simulink model "channel_rayleigh"  (R2020a)
settings: Solver=ode45  StartTime=0.0  StopTime=10.0  RelTol=1e-3  EnableMultiTasking=on
libraries: commdigbbndpm3 x2, commsink2 x1
settings Model: Creator=Csurgai  LastModifiedBy=L.Csurgai
settings DataIOCC: LimitDataPoints=on  SaveFormat=Array  SignalLoggingSaveFormat=ModelDataLogs  ReturnWorkspaceOutputs=off
settings OptimizationCC: InitFltsAndDblsToZero=on  LifeSpan=inf
settings DebuggingCC: SaveWithParameterizedLinksMsg=none  UnderspecifiedInitializationDetection=Classic  MergeDetectMultiDrivingBlocksExec=none  SignalResolutionControl=TryResolveAllWithWarning  SolverPrmCheckMsg=warning  MultiTaskDSMMsg=warning  MultiTaskCondExecSysMsg=none  FcnCallInpInsideContextMsg=warning  SFUnexpectedBacktrackingDiag=warning  SFNoUnconditionalDefaultTransitionDiag=warning  SFExecutionAtInitializationDiag=none  ArithmeticOperatorsInVariantConditions=warning
settings HardwareCC: ProdBitPerPointer=32  ProdBitPerSizeT=32  ProdBitPerPtrDiffT=32  ProdLargestAtomicFloat=None  ProdIntDivRoundTo=Undefined  ProdEndianess=Unspecified  ProdWordSize=32  ProdHWDeviceType=32-bit Generic
settings ModelReferenceCC: PropagateSignalLabelsOutOfModel=off
settings SFSimCC: SimUseLocalCustomCode=off  CustomCodeUndefinedFunction=UseInterfaceOnly
settings RTWCC: RTWUseLocalCustomCode=off
settings CodeAppCC: StateflowObjectComments=on
settings GRTTargetCC: TargetFcnLib=ansi_tfl_tmw.mat  TargetLangStandard=C89/C90 (ANSI)  CombineOutputUpdateFcns=off  GRTInterface=on
settings ConfigComp: CovMetricSettings=dw  CovHtmlReporting=on  CovSaveCumulativeToWorkspaceVar=on  CovSaveSingleToWorkspaceVar=on  CovExternalEMLEnable=off

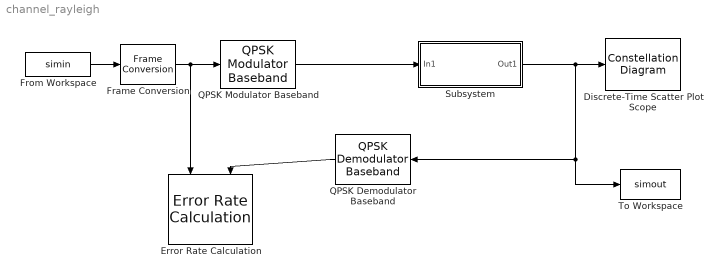
== system channel_rayleigh ==
  Discrete-Time Scatter Plot Scope : ConstellationDiagram  Tag=ScatterPlot
  Error Rate Calculation : commsink2/Error Rate Calculation  N=0  st_delay=0  cp_mode=Entire frame  subframe=[]  PMode=Workspace  WsName=ErrorVec  RsMode2=off  stop=off  numErr=100  maxBits=1e6
  Frame Conversion : FrameConversion
  From Workspace : FromWorkspace  VariableName=simin  SampleTime=1e-3
  QPSK Demodulator Baseband : commdigbbndpm3/QPSK Demodulator Baseband  OutType=Integer  DecType=Hard decision  VarSource=Dialog  Variance=1  Dec=Binary  Ph=pi/4  outDtype1=double  outDtype2=double  derotateFactorWordLen=16  derotateFactorDataTypeStr=Inherit: Same word length as input  derotateFactorLastDataTypeStr=Inherit: Same word length as input
  QPSK Modulator Baseband : commdigbbndpm3/QPSK Modulator Baseband  InType=Integer  Enc=Binary  Ph=pi/4  outDtype=double  outWordLen=16  outUDDataType=sfix(16)  outFracLenMode=Best precision  outFracLen=15  outDataTypeStr=double  outLastDataTypeStr=double
  Subsystem : Subsystem
  To Workspace : ToWorkspace  VariableName=simout  SaveFormat=Structure  SampleTime=-1
      settings: Save2DSignal=2-D array (concatenate along first dimension)
  wires:
  From Workspace/1 -> Frame Conversion/1
  Frame Conversion/1 -> QPSK Modulator Baseband/1, Error Rate Calculation/1
  QPSK Demodulator Baseband/1 -> Error Rate Calculation/2
  QPSK Modulator Baseband/1 -> Subsystem/1(In1)
  Subsystem/1(Out1) -> Discrete-Time Scatter Plot Scope/1, To Workspace/1, QPSK Demodulator Baseband/1

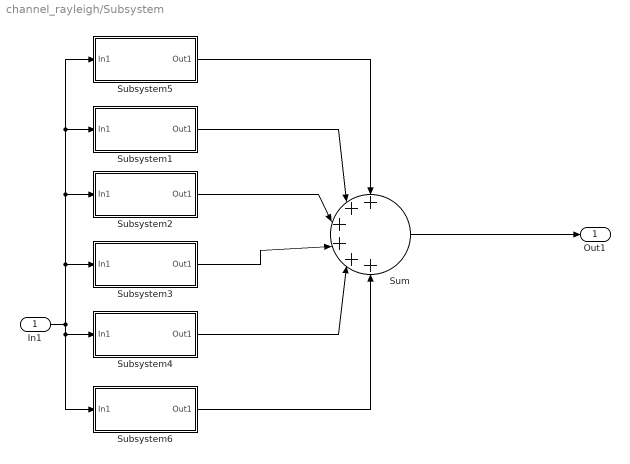
== system channel_rayleigh/Subsystem ==
  In1 : Inport
  Subsystem1 : Subsystem
  Subsystem2 : Subsystem
  Subsystem3 : Subsystem
  Subsystem4 : Subsystem
  Subsystem5 : Subsystem
  Subsystem6 : Subsystem
  Sum : Sum  Inputs=++++++
  Out1 : Outport
  wires:
  Sum/1 -> Out1/1
  Subsystem5/1(Out1) -> Sum/1
  Subsystem1/1(Out1) -> Sum/2
  Subsystem2/1(Out1) -> Sum/3
  Subsystem3/1(Out1) -> Sum/4
  Subsystem4/1(Out1) -> Sum/5
  Subsystem6/1(Out1) -> Sum/6
  In1/1 -> Subsystem5/1(In1), Subsystem1/1(In1), Subsystem2/1(In1), Subsystem3/1(In1), Subsystem6/1(In1), Subsystem4/1(In1)

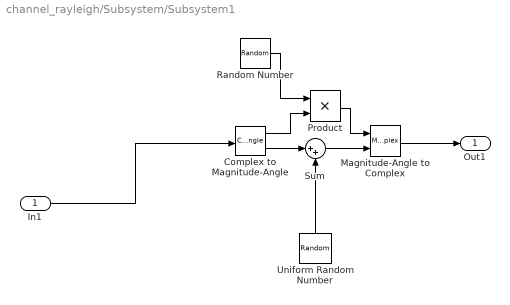
== system channel_rayleigh/Subsystem/Subsystem1 ==
  In1 : Inport
  Complex to Magnitude-Angle : ComplexToMagnitudeAngle  SampleTime=1e-3
  Magnitude-Angle to Complex : MagnitudeAngleToComplex
  Product : Product  RndMeth=Zero
  Random Number : RandomNumber  Mean=.8  Variance=.1  Seed=randi(2e5)  SampleTime=1e-3
  Sum : Sum  Inputs=|++
  Uniform Random Number : UniformRandomNumber  Minimum=0  Maximum=pi  Seed=randi(2e5)  SampleTime=1e-3
  Out1 : Outport
  wires:
  Magnitude-Angle to Complex/1 -> Out1/1
  Complex to Magnitude-Angle/2 -> Sum/1
  Sum/1 -> Magnitude-Angle to Complex/2
  Uniform Random Number/1 -> Sum/2
  In1/1 -> Complex to Magnitude-Angle/1
  Complex to Magnitude-Angle/1 -> Product/2
  Random Number/1 -> Product/1
  Product/1 -> Magnitude-Angle to Complex/1

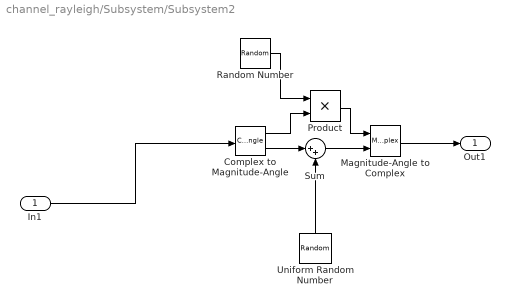
== system channel_rayleigh/Subsystem/Subsystem2 ==
  In1 : Inport
  Complex to Magnitude-Angle : ComplexToMagnitudeAngle  SampleTime=1e-3
  Magnitude-Angle to Complex : MagnitudeAngleToComplex
  Product : Product  RndMeth=Zero
  Random Number : RandomNumber  Mean=.7  Variance=.1  Seed=randi(2e5)  SampleTime=1e-3
  Sum : Sum  Inputs=|++
  Uniform Random Number : UniformRandomNumber  Minimum=0  Maximum=pi  Seed=randi(2e5)  SampleTime=1e-3
  Out1 : Outport
  wires:
  Magnitude-Angle to Complex/1 -> Out1/1
  Complex to Magnitude-Angle/2 -> Sum/1
  Sum/1 -> Magnitude-Angle to Complex/2
  Uniform Random Number/1 -> Sum/2
  In1/1 -> Complex to Magnitude-Angle/1
  Complex to Magnitude-Angle/1 -> Product/2
  Random Number/1 -> Product/1
  Product/1 -> Magnitude-Angle to Complex/1

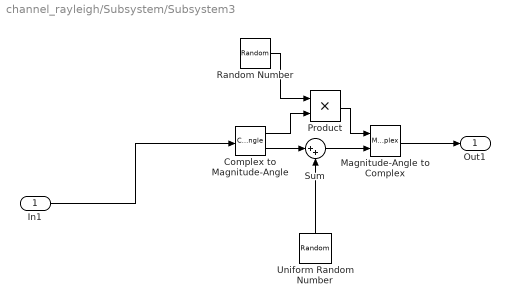
== system channel_rayleigh/Subsystem/Subsystem3 ==
  In1 : Inport
  Complex to Magnitude-Angle : ComplexToMagnitudeAngle  SampleTime=1e-3
  Magnitude-Angle to Complex : MagnitudeAngleToComplex
  Product : Product  RndMeth=Zero
  Random Number : RandomNumber  Mean=.85  Variance=.1  Seed=randi(2e5)  SampleTime=1e-3
  Sum : Sum  Inputs=|++
  Uniform Random Number : UniformRandomNumber  Minimum=0  Maximum=pi  Seed=randi(2e5)  SampleTime=1e-3
  Out1 : Outport
  wires:
  Magnitude-Angle to Complex/1 -> Out1/1
  Complex to Magnitude-Angle/2 -> Sum/1
  Sum/1 -> Magnitude-Angle to Complex/2
  Uniform Random Number/1 -> Sum/2
  In1/1 -> Complex to Magnitude-Angle/1
  Complex to Magnitude-Angle/1 -> Product/2
  Random Number/1 -> Product/1
  Product/1 -> Magnitude-Angle to Complex/1

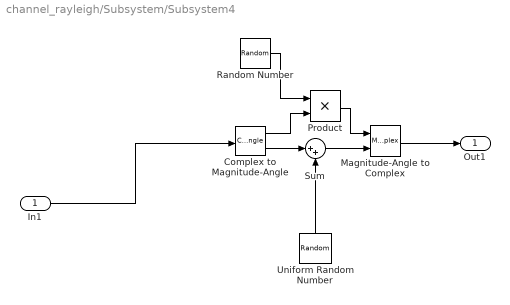
== system channel_rayleigh/Subsystem/Subsystem4 ==
  In1 : Inport
  Complex to Magnitude-Angle : ComplexToMagnitudeAngle  SampleTime=1e-3
  Magnitude-Angle to Complex : MagnitudeAngleToComplex
  Product : Product  RndMeth=Zero
  Random Number : RandomNumber  Mean=.9  Variance=.1  Seed=randi(2e5)  SampleTime=1e-3
  Sum : Sum  Inputs=|++
  Uniform Random Number : UniformRandomNumber  Minimum=0  Maximum=pi  Seed=randi(2e5)  SampleTime=1e-3
  Out1 : Outport
  wires:
  Magnitude-Angle to Complex/1 -> Out1/1
  Complex to Magnitude-Angle/2 -> Sum/1
  Sum/1 -> Magnitude-Angle to Complex/2
  Uniform Random Number/1 -> Sum/2
  In1/1 -> Complex to Magnitude-Angle/1
  Complex to Magnitude-Angle/1 -> Product/2
  Random Number/1 -> Product/1
  Product/1 -> Magnitude-Angle to Complex/1

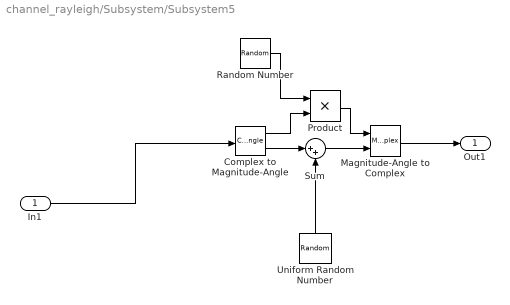
== system channel_rayleigh/Subsystem/Subsystem5 ==
  In1 : Inport
  Complex to Magnitude-Angle : ComplexToMagnitudeAngle  SampleTime=1e-3
  Magnitude-Angle to Complex : MagnitudeAngleToComplex
  Product : Product  RndMeth=Zero
  Random Number : RandomNumber  Mean=.6  Variance=.1  Seed=randi(2e5)  SampleTime=1e-3
  Sum : Sum  Inputs=|++
  Uniform Random Number : UniformRandomNumber  Minimum=0  Maximum=pi  Seed=randi(2e5)  SampleTime=1e-3
  Out1 : Outport
  wires:
  Magnitude-Angle to Complex/1 -> Out1/1
  Complex to Magnitude-Angle/2 -> Sum/1
  Sum/1 -> Magnitude-Angle to Complex/2
  Uniform Random Number/1 -> Sum/2
  In1/1 -> Complex to Magnitude-Angle/1
  Complex to Magnitude-Angle/1 -> Product/2
  Random Number/1 -> Product/1
  Product/1 -> Magnitude-Angle to Complex/1

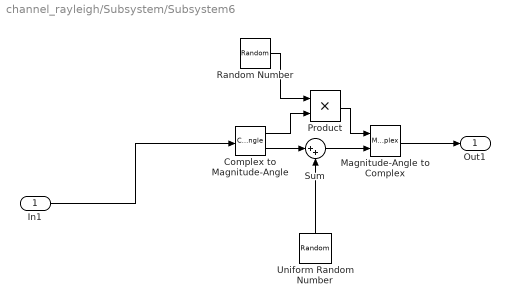
== system channel_rayleigh/Subsystem/Subsystem6 ==
  In1 : Inport
  Complex to Magnitude-Angle : ComplexToMagnitudeAngle  SampleTime=1e-3
  Magnitude-Angle to Complex : MagnitudeAngleToComplex
  Product : Product  RndMeth=Zero
  Random Number : RandomNumber  Mean=.8  Variance=.1  Seed=randi(2e5)  SampleTime=1e-3
  Sum : Sum  Inputs=|++
  Uniform Random Number : UniformRandomNumber  Minimum=0  Maximum=pi  Seed=randi(2e5)  SampleTime=1e-3
  Out1 : Outport
  wires:
  Magnitude-Angle to Complex/1 -> Out1/1
  Complex to Magnitude-Angle/2 -> Sum/1
  Sum/1 -> Magnitude-Angle to Complex/2
  Uniform Random Number/1 -> Sum/2
  In1/1 -> Complex to Magnitude-Angle/1
  Complex to Magnitude-Angle/1 -> Product/2
  Random Number/1 -> Product/1
  Product/1 -> Magnitude-Angle to Complex/1
